simulink model "modelo_SEIRV"  (R2019b)
settings: Solver=VariableStepAuto  StartTime=0.0  StopTime=365  RelTol=1e-3
undefined symbols (not defined in the file): beta, E0, gamma, I0, nu, R0, S0, sigma
settings Model: Creator=lucia  LastModifiedBy=lucia

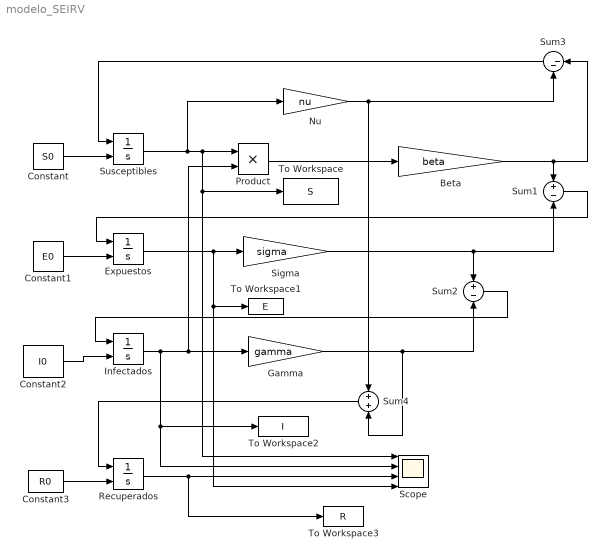
== system modelo_SEIRV ==
  Beta : Gain  Gain=beta
  Constant : Constant  Value=S0
  Constant1 : Constant  Value=E0
  Constant2 : Constant  Value=I0
  Constant3 : Constant  Value=R0
  Expuestos : Integrator  InitialConditionSource=external
  Gamma : Gain  Gain=gamma
  Infectados : Integrator  InitialConditionSource=external
  Nu : Gain  Gain=nu
  Product : Product
  Recuperados : Integrator  InitialConditionSource=external
  Scope : Scope  NumInputPorts=4
  Sigma : Gain  Gain=sigma
  Sum1 : Sum  Inputs=+-
  Sum2 : Sum  Inputs=+-
  Sum3 : Sum  Inputs=|--
  Sum4 : Sum
  Susceptibles : Integrator  InitialConditionSource=external
  To Workspace : ToWorkspace  VariableName=S  SaveFormat=Structure With Time  SampleTime=-1
  To Workspace1 : ToWorkspace  VariableName=E  SaveFormat=Structure With Time  SampleTime=-1
  To Workspace2 : ToWorkspace  VariableName=I  SaveFormat=Structure With Time  SampleTime=-1
  To Workspace3 : ToWorkspace  VariableName=R  SaveFormat=Structure With Time  SampleTime=-1
  wires:
  Sigma/1 -> Sum1/2, Sum2/1
  Recuperados/1 -> To Workspace3/1, Scope/3
  Gamma/1 -> Sum2/2, Sum4/2
  Constant/1 -> Susceptibles/2
  Sum1/1 -> Expuestos/1
  Sum3/1 -> Susceptibles/1
  Sum2/1 -> Infectados/1
  Susceptibles/1 -> Nu/1, To Workspace/1, Scope/1, Product/1
  Product/1 -> Beta/1
  Constant2/1 -> Infectados/2
  Constant1/1 -> Expuestos/2
  Infectados/1 -> Scope/2, To Workspace2/1, Product/2, Gamma/1
  Beta/1 -> Sum3/1, Sum1/1
  Expuestos/1 -> To Workspace1/1, Scope/4, Sigma/1
  Constant3/1 -> Recuperados/2
  Nu/1 -> Sum3/2, Sum4/1
  Sum4/1 -> Recuperados/1
